simulink model "try_case4"  (R2015b)
settings: Solver=FixedStepAuto  StartTime=12  StopTime=123.2400  FixedStep=0.02  RelTol=1e-3
values from neighbouring files (symbols this model uses):
  kg = b(j)    [Num4s.m]    (also in cont.m; kg_ko.mat = 0.039; num4_45deg.m = b(i); sys4_mass.m)
libraries: simulink x1
settings Model: Creator=guilh_000  LastModifiedBy=guilh_000

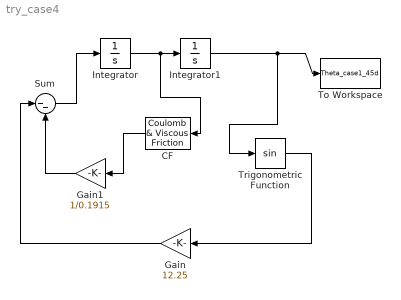
== system try_case4 ==
  CF : simulink/Discontinuities/Coulomb & Viscous Friction  offset=ko  gain=kg
  Gain : Gain  Gain=12.25
  Gain1 : Gain  Gain=1/0.1915
  Integrator : Integrator
  Integrator1 : Integrator  InitialCondition=-pi/4
  Sum : Sum  Inputs=|--
  To Workspace : ToWorkspace  VariableName=Theta_case1_45d  SampleTime=-1
  Trigonometric Function : Trigonometry
  wires:
  Integrator/1 -> CF/1, Integrator1/1
  Integrator1/1 -> Trigonometric Function/1, To Workspace/1
  Trigonometric Function/1 -> Gain/1
  Gain/1 -> Sum/1
  Sum/1 -> Integrator/1
  CF/1 -> Gain1/1
  Gain1/1 -> Sum/2
